simulink model "NM_v4_GUI"  (R2024b)
settings: Solver=FixedStepAuto  StartTime=0.0  StopTime=solvertime  FixedStep=stepsize  RelTol=1e-3
undefined symbols (not defined in the file or in its folder): phase_delay, pulse_amp, pulse_rate
libraries: Libs_unified x1
settings Model: Creator=ball907  LastModifiedBy=ball907

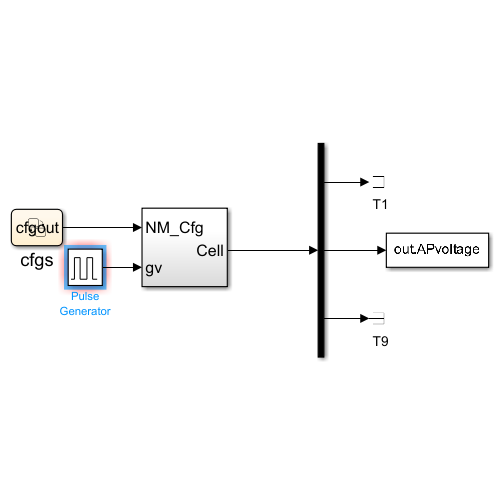
[thumbnail: Simulink's stored preview of the top-level diagram]
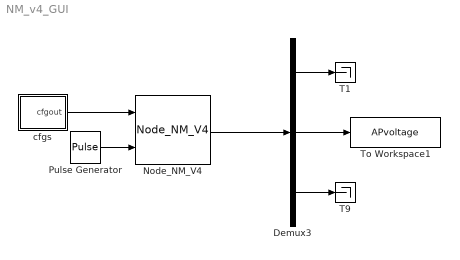
== system NM_v4_GUI ==
  Demux3 : Demux  Outputs=[1, 1, 3]
  Node_NM_V4 : Libs_unified/Node_NM_V4  SystemSampleTime=-1  VariantActivationTime=update diagram  AllowFlexibleInterface=on  Latency=0  AutoFrameSizeCalculation=off
  Pulse Generator : DiscretePulseGenerator  PulseType=Time based  Amplitude=pulse_amp  Period=pulse_rate  PhaseDelay=phase_delay
  T1 : Terminator
  T9 : Terminator
  To Workspace1 : ToWorkspace  VariableName=APvoltage  SaveFormat=Timeseries  SampleTime=-1
  cfgs : Stateflow chart  TreatAsAtomicUnit=on
  wires:
  Demux3/3 -> T9/1
  Node_NM_V4/1 -> Demux3/1
  Demux3/2 -> To Workspace1/1
  Pulse Generator/1 -> Node_NM_V4/2
  cfgs/1(cfgout) -> Node_NM_V4/1
  Demux3/1 -> T1/1

== stateflow chart NM_v4_GUI/cfgs ==
  settings: executeAtInitialization=1
  state Ini
  (default) -> Ini : {cfgout=auto;}
  data: cfg function_output; params parameter; cfgout output
  function cfg = auto:
    | function cfg = auto
    | 
    | BCL=params(1,1);
    | SD=params(1,2);
    | f1=params(1,3);
    | f2=params(1,4);
    | sigma1sq=params(1,5);
    | sigma2sq=params(1,6);
    | 
    | d2=params(1,7); 
    | erp_out=params(1,8);
    | d0=params(1,9); 
    | MDP=params(1,10);
    | VT_N=params(1,11); 
    | VR_N=params(1,12); 
    | Vh_out=params(1,13);
    | 
    | hr_out=params(1,14); 
    | hs_out=params(1,15);
    | s_out=params(1,16);
    | j_out=params(1,17);
    | m_out=params(1,18); 
    | 
    | h_out=params(1,19);
    | f_out=params(1,20);
    | 
    | r_out=params(1,21);
    | 
    | ax0=params(1,22);
    | ay0=params(1,23);
    | az0=params(1,24);
    |  
    | ax1=params(1,25);
    | ay1=params(1,26);
    | az1=params(1,27);
    |  
    | ax2=params(1,28);
    | ay2=params(1,29);
    | az2=params(1,30);
    |  
    | ax3=params(1,31);
    | ay3=params(1,32);
    | az3=params(1,33);
    |  
    | bx1=params(1,34);
    | by1=params(1,35);
    | bz1=params(1,36);
    | 
    | VR_M=params(1,37);
    | VT_M=params(1,38);
    | VO=params(1,39);
    |  
    | a=params(1,40);
    | b=params(1,41);
    | c=params(1,42);
    | d=params(1,43);
    | e=params(1,44);
    | x=params(1,45);
    | y=params(1,46);
    | 
    | Dij=params(1,47);
    | Dji=params(1,48);
    | 
    | 
    | cfg=[BCL, SD, f1,f2,sigma1sq, sigma2sq,d2,erp_out,d0,MDP,VT_N,VR_N,Vh_out,hr_out,hs_out,s_out,j_out,m_out,h_out,f_out,r_out,x,y,ax0,ay0,az0,ax1,ay1,az1,ax2,ay2,az2,ax3,ay3,az3,bx1,by1,bz1,VR_M,VT_M,VO,a,b,c,d,e,x,y,Dij,Dji];
    | end
